simulink model "ANNA"  (R2021a)
settings: Solver=VariableStepAuto  StartTime=0.0  StopTime=10.0  RelTol=1e-3
libraries: fl_lib x18, nesl_utility x7, ee_lib x5
settings Model: Creator=BenjaminAtadana  LastModifiedBy=BenjaminAtadana

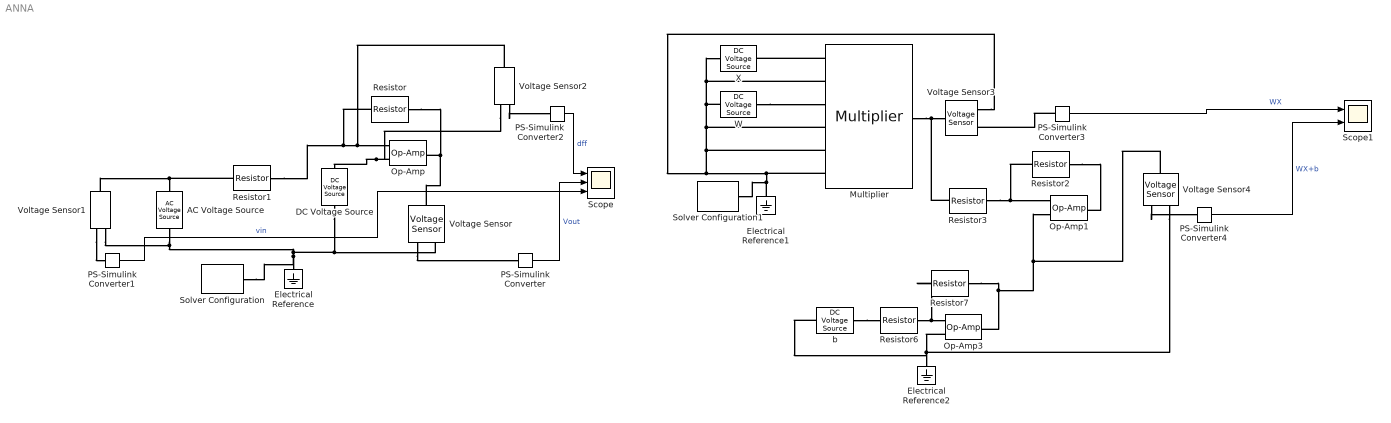
== system ANNA ==
  AC Voltage Source : fl_lib/Electrical/Electrical Sources/AC Voltage Source  amp=5 V  shift=0 deg  frequency=0.3 Hz  omega=0 rad/s
  DC Voltage Source : ee_lib/Additional Components/SPICE Sources/DC Voltage Source  DC=2 V
  Electrical Reference : fl_lib/Electrical/Electrical Elements/Electrical Reference
  Electrical Reference1 : fl_lib/Electrical/Electrical Elements/Electrical Reference
  Electrical Reference2 : fl_lib/Electrical/Electrical Elements/Electrical Reference
  Multiplier : ee_lib/Integrated Circuits/Multiplier  K=1 V  A=1  Rin=10e6 Ohm  Vdiff=10 V  Rout=0.1 Ohm  Vmin=-11 V  Vmax=11 V  Vdotmax=20 V/us  f=1 MHz  V0=0 V
      settings: SourceProductBaseCode=PS  InternalSimscapePortConfiguration="{\"Bottom\":[],\"Left\":[{\"id\":\"X1\",\"label\":\"X1\",\"type\":\"foundation.electrical.electrical\"},{\"id\":\"X2\",\"label\":\"X2\",\"type\":\"foundation.electrical.electrical\"},{\"id\":\"Y1\",\"label\":\"Y1\",\"type\":\"foundation.electrical.electrical\"},{\"id\":\"Y2\",\"label\":\"Y2\",\"type\":\"foundation.electrical.electrical\"},{\"id\":\"Z1\",\"label\":\"Z1\",\"type\":\"foundation.electrical.electrical\"},{\"id\":\"Z2\",\"label\":\"Z2\",\"type\":\"foundation.electrical.electrical\"}],\"Right\":[{\"id\":\"out\",\"label\":\"\",\"type\":\"foundation.electrical.electrical\"}],\"Top\":[]}"
  Op-Amp : fl_lib/Electrical/Electrical Elements/Op-Amp  outI_specify=off  outI_priority=None  outI=0 A  outI_nominal_specify=off  outI_nominal_unit=A  outI_nominal_value=1
  Op-Amp1 : fl_lib/Electrical/Electrical Elements/Op-Amp  outI_specify=off  outI_priority=None  outI=0 A  outI_nominal_specify=off  outI_nominal_unit=A  outI_nominal_value=1
  Op-Amp3 : fl_lib/Electrical/Electrical Elements/Op-Amp  outI_specify=off  outI_priority=None  outI=0 A  outI_nominal_specify=off  outI_nominal_unit=A  outI_nominal_value=1
  PS-Simulink Converter{,1..4} (5 alike) : nesl_utility/PS-Simulink Converter  PhysicalDomain=network_engine_domain  SubClassName=ps_output  LeftPortType=input  RightPortType=output  PseudoPeriodic=off  Frequencies=[]  Unit=inherit  AffineConversion=off
      settings: SourceProductBaseCode=PW,SS
  Resistor{,2..3,6..7} (5 alike) : fl_lib/Electrical/Electrical Elements/Resistor  R=10 Ohm  i_specify=off  i_priority=None  i=0 A  i_nominal_specify=off  i_nominal_unit=A  i_nominal_value=1  v_specify=off  v_priority=None  v=0 V  v_nominal_specify=off  v_nominal_unit=V  v_nominal_value=1
  Resistor1 : fl_lib/Electrical/Electrical Elements/Resistor  R=2 Ohm  i_specify=off  i_priority=None  i=0 A  i_nominal_specify=off  i_nominal_unit=A  i_nominal_value=1  v_specify=off  v_priority=None  v=0 V  v_nominal_specify=off  v_nominal_unit=V  v_nominal_value=1
  Scope : Scope  NumInputPorts=3
  Scope1 : Scope  NumInputPorts=2
  Solver Configuration : nesl_utility/Solver Configuration  PhysicalDomain=network_engine_domain  SubClassName=solver  LeftPortType=input  RightPortType=generic  Tones=[]  Harmonics=[]  SimulateNoise=off  Profile=off  UseLocalSampling=off  EnableSwitchedLinearOptims=on  FrequencyDomain=off  UseCCode=off  RelTol=0.001  AbsTol=1e-06  MinStep=1e-09  ToWorkspace=off  RevertToSquareIcSolve=off  NumHomotopyIterations=100  PhasorMode=off  PhasorModeNumHarmonics=1  DoDC=off  ResidualTolerance=1e-09  UseLocalSolver=off  LocalSolverChoice=NE_BACKWARD_EULER_ADVANCER  LocalSolverSampleTime=0.001  DoFixedCost=off  MaxNonlinIter=3  MaxModeIter=2  ComputeImpulses=off  ImpulseIterations=2  LinearAlgebra=auto  EquationFormulation=NE_TIME_EF  DelaysMemoryBudget=1024  AutomaticFiltering=on  FilteringTimeConstant=0.001  PartitionStorageMethod=AS_NEEDED  PartitionMemoryBudget=1024  PartitionMethod=ROBUST
      settings: SourceProductBaseCode=PW,SS
  Solver Configuration1 : nesl_utility/Solver Configuration  PhysicalDomain=network_engine_domain  SubClassName=solver  LeftPortType=input  RightPortType=generic  Tones=[]  Harmonics=[]  SimulateNoise=off  Profile=off  UseLocalSampling=off  EnableSwitchedLinearOptims=on  FrequencyDomain=off  UseCCode=off  RelTol=0.001  AbsTol=1e-06  MinStep=1e-09  ToWorkspace=off  RevertToSquareIcSolve=off  NumHomotopyIterations=100  PhasorMode=off  PhasorModeNumHarmonics=1  DoDC=off  ResidualTolerance=1e-09  UseLocalSolver=off  LocalSolverChoice=NE_BACKWARD_EULER_ADVANCER  LocalSolverSampleTime=0.001  DoFixedCost=off  MaxNonlinIter=3  MaxModeIter=2  ComputeImpulses=off  ImpulseIterations=2  LinearAlgebra=auto  EquationFormulation=NE_TIME_EF  DelaysMemoryBudget=1024  AutomaticFiltering=on  FilteringTimeConstant=0.001  PartitionStorageMethod=AS_NEEDED  PartitionMemoryBudget=1024  PartitionMethod=ROBUST
      settings: SourceProductBaseCode=PW,SS
  Voltage Sensor{,1..4} (5 alike) : fl_lib/Electrical/Electrical Sensors/Voltage Sensor
  W : ee_lib/Additional Components/SPICE Sources/DC Voltage Source  DC=2 V
  X : ee_lib/Additional Components/SPICE Sources/DC Voltage Source  DC=2 V
  b : ee_lib/Additional Components/SPICE Sources/DC Voltage Source  DC=2 V
  wires:
  PS-Simulink Converter/1 -> Scope/2  "Vout"
  PS-Simulink Converter1/1 -> Scope/3  "vin"
  PS-Simulink Converter2/1 -> Scope/1  "dff"
  PS-Simulink Converter3/1 -> Scope1/1  "WX"
  PS-Simulink Converter4/1 -> Scope1/2  "WX+b"
  connections:
  Resistor1/RConn1 -- Resistor/LConn1 -- Op-Amp/LConn2 -- Voltage Sensor2/LConn1
  Resistor1/LConn1 -- Voltage Sensor1/LConn1 -- AC Voltage Source/LConn1
  AC Voltage Source/RConn1 -- Voltage Sensor1/RConn2 -- DC Voltage Source/RConn1 -- Voltage Sensor/RConn2 -- Solver Configuration/RConn1 -- Electrical Reference/LConn1
  Resistor/RConn1 -- Voltage Sensor/LConn1 -- Op-Amp/RConn1
  Voltage Sensor/RConn1 -- PS-Simulink Converter/LConn1
  Voltage Sensor1/RConn1 -- PS-Simulink Converter1/LConn1
  Op-Amp/LConn1 -- Voltage Sensor2/RConn2 -- DC Voltage Source/LConn1
  Voltage Sensor2/RConn1 -- PS-Simulink Converter2/LConn1
  Multiplier/LConn1 -- X/LConn1
  W/LConn1 -- Multiplier/LConn3
  Multiplier/LConn2 -- Solver Configuration1/RConn1 -- Electrical Reference1/LConn1 -- Multiplier/LConn6 -- Voltage Sensor3/RConn2 -- Multiplier/LConn5 -- Multiplier/LConn4 -- W/RConn1 -- X/RConn1
  Multiplier/RConn1 -- Resistor3/LConn1 -- Voltage Sensor3/LConn1
  PS-Simulink Converter3/LConn1 -- Voltage Sensor3/RConn1
  Resistor3/RConn1 -- Resistor2/LConn1 -- Op-Amp1/LConn1
  Resistor2/RConn1 -- Op-Amp1/RConn1
  Resistor7/RConn1 -- Op-Amp3/RConn1 -- Voltage Sensor4/LConn1 -- Op-Amp1/LConn2
  Resistor6/RConn1 -- Resistor7/LConn1 -- Op-Amp3/LConn2
  b/LConn1 -- Resistor6/LConn1
  Op-Amp3/LConn1 -- Voltage Sensor4/RConn2 -- b/RConn1 -- Electrical Reference2/LConn1
  Voltage Sensor4/RConn1 -- PS-Simulink Converter4/LConn1
